simulink library "csu_imk_imu_kinematics_lib_a"  (R2014b)
settings: Solver=ode45  SolverMode=SingleTasking  StartTime=0.0  StopTime=10.0  RelTol=1e-3
undefined symbols (not defined in the file or in its folder): imu_dcm, imu_position
libraries: util_common_lib x3, util_quat_lib x3, util_info_lib x1
settings Model: Creator=hcannon  LastModifiedBy=mstewart

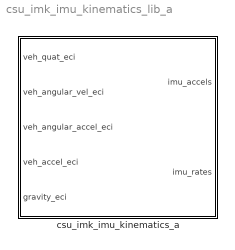
== system csu_imk_imu_kinematics_lib_a ==
  csu_imk_imu_kinematics_a : Subsystem

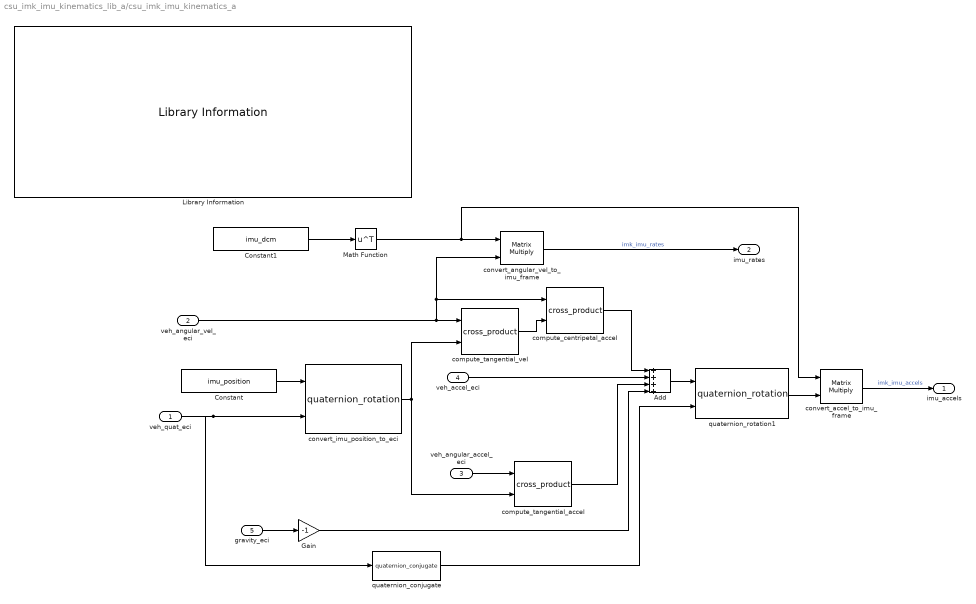
== system csu_imk_imu_kinematics_lib_a/csu_imk_imu_kinematics_a ==
  veh_quat_eci : Inport
  veh_angular_vel_eci : Inport  Port=2
  veh_angular_accel_eci : Inport  Port=3
  veh_accel_eci : Inport  Port=4
  gravity_eci : Inport  Port=5
  Add : Sum  Inputs=++++
  Constant : Constant  Value=imu_position
  Constant1 : Constant  Value=imu_dcm  VectorParams1D=off
  Gain : Gain  Gain=-1
  Library Information : util_info_lib/Library Information  owner='NONE'
  Math Function : Math  Operator=transpose  SaturateOnIntegerOverflow=on
  compute_centripetal_accel : util_common_lib/cross_product  SystemSampleTime=-1
  compute_tangential_accel : util_common_lib/cross_product  SystemSampleTime=-1
  compute_tangential_vel : util_common_lib/cross_product  SystemSampleTime=-1
  convert_accel_to_imu_frame : Product  Multiplication=Matrix(*)  RndMeth=Zero
  convert_angular_vel_to_imu_frame : Product  Multiplication=Matrix(*)  RndMeth=Zero
  convert_imu_position_to_eci : util_quat_lib/quaternion_rotation  SystemSampleTime=-1
  quaternion_conjugate : util_quat_lib/quaternion_conjugate  SystemSampleTime=-1
  quaternion_rotation1 : util_quat_lib/quaternion_rotation  SystemSampleTime=-1
  imu_accels : Outport
  imu_rates : Outport  Port=2
  wires:
  Constant/1 -> convert_imu_position_to_eci/1
  quaternion_rotation1/1 -> convert_accel_to_imu_frame/2
  convert_angular_vel_to_imu_frame/1 -> imu_rates/1  "imk_imu_rates"
  convert_accel_to_imu_frame/1 -> imu_accels/1  "imk_imu_accels"
  Constant1/1 -> Math Function/1
  Add/1 -> quaternion_rotation1/1
  Gain/1 -> Add/4
  gravity_eci/1 -> Gain/1
  compute_tangential_accel/1 -> Add/3
  compute_centripetal_accel/1 -> Add/1
  compute_tangential_vel/1 -> compute_centripetal_accel/2
  veh_angular_vel_eci/1 -> convert_angular_vel_to_imu_frame/2, compute_centripetal_accel/1, compute_tangential_vel/1
  veh_angular_accel_eci/1 -> compute_tangential_accel/1
  convert_imu_position_to_eci/1 -> compute_tangential_vel/2, compute_tangential_accel/2
  veh_quat_eci/1 -> quaternion_conjugate/1, convert_imu_position_to_eci/2
  Math Function/1 -> convert_accel_to_imu_frame/1, convert_angular_vel_to_imu_frame/1
  veh_accel_eci/1 -> Add/2
  quaternion_conjugate/1 -> quaternion_rotation1/2
